simulink model "Lab07B"  (R2021a)
settings: Solver=VariableStepAuto  StartTime=0.0  StopTime=50  RelTol=1e-3
undefined symbols (not defined in the file or in its folder): Kh, Kv
libraries: simulink x1
settings Model: Creator=levivandek  LastModifiedBy=levivandek

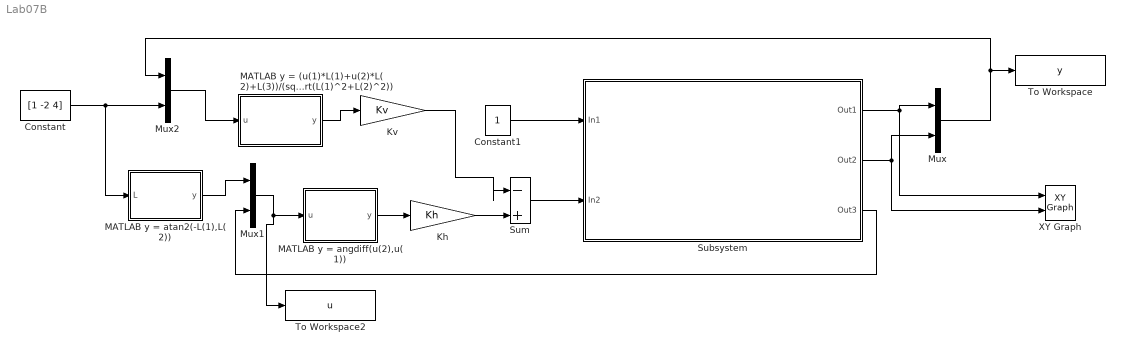
== system Lab07B ==
  Constant : Constant  Value=[1 -2 4]
  Constant1 : Constant
  Kh : Gain  Gain=Kh
  Kv : Gain  Gain=Kv
  MATLAB y = (u(1)*L(1)+u(2)*L(2)+L(3))/(sqrt(L(1)^2+L(2)^2)) : MATLAB Function  TreatAsAtomicUnit=on
  MATLAB y = angdiff(u(2),u(1)) : MATLAB Function  TreatAsAtomicUnit=on
  MATLAB y = atan2(-L(1),L(2)) : MATLAB Function  TreatAsAtomicUnit=on
  Mux : Mux  Inputs=2
  Mux1 : Mux  Inputs=2
  Mux2 : Mux  Inputs=2
  Subsystem : Subsystem
  Sum : Sum  Inputs=|-+
  To Workspace : ToWorkspace  VariableName=y  SaveFormat=Timeseries  SampleTime=-1
  To Workspace2 : ToWorkspace  VariableName=u  SaveFormat=Timeseries  SampleTime=-1
  XY Graph : simulink/Sinks/XY Graph  xmin=-10  xmax=10  ymin=-4  ymax=12  st=-1
  wires:
  Subsystem/2(Out2) -> Mux/2, XY Graph/2
  Subsystem/1(Out1) -> XY Graph/1, Mux/1
  Mux/1 -> Mux2/1, To Workspace/1
  Subsystem/3(Out3) -> Mux1/2
  MATLAB y = angdiff(u(2),u(1))/1(y) -> Kh/1
  Mux1/1 -> To Workspace2/1, MATLAB y = angdiff(u(2),u(1))/1(u)
  MATLAB y = (u(1)*L(1)+u(2)*L(2)+L(3))/(sqrt(L(1)^2+L(2)^2))/1(y) -> Kv/1
  MATLAB y = atan2(-L(1),L(2))/1(y) -> Mux1/1
  Constant/1 -> MATLAB y = atan2(-L(1),L(2))/1(L), Mux2/2
  Kh/1 -> Sum/2
  Kv/1 -> Sum/1
  Sum/1 -> Subsystem/2(In2)
  Constant1/1 -> Subsystem/1(In1)
  Mux2/1 -> MATLAB y = (u(1)*L(1)+u(2)*L(2)+L(3))/(sqrt(L(1)^2+L(2)^2))/1(u)

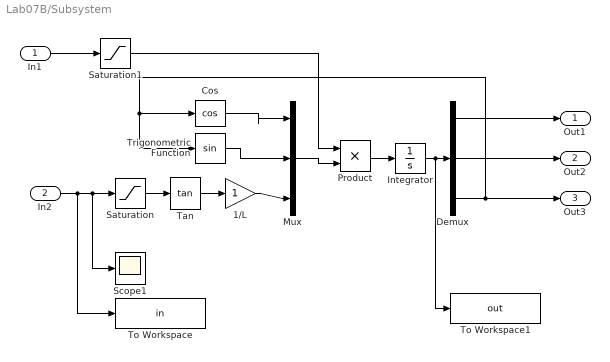
== system Lab07B/Subsystem ==
  In1 : Inport
  In2 : Inport  Port=2
  1/L : Gain
  Cos : Trigonometry  Operator=cos
  Demux : Demux  Outputs=3
  Integrator : Integrator  InitialCondition=[8 5 pi/2]
  Mux : Mux  Inputs=3
  Product : Product
  Saturation : Saturate  UpperLimit=1  LowerLimit=-1
  Saturation1 : Saturate  UpperLimit=1  LowerLimit=-1
  Scope1 : Scope
  Tan : Trigonometry  Operator=tan
  To Workspace : ToWorkspace  VariableName=in  SaveFormat=Timeseries  SampleTime=-1
  To Workspace1 : ToWorkspace  VariableName=out  SaveFormat=Timeseries  SampleTime=-1
  Trigonometric Function : Trigonometry
  Out1 : Outport
  Out2 : Outport  Port=2
  Out3 : Outport  Port=3
  wires:
  Cos/1 -> Mux/1
  Demux/1 -> Out1/1
  In2/1 -> To Workspace/1, Scope1/1, Saturation/1
  1/L/1 -> Mux/3
  Product/1 -> Integrator/1
  Integrator/1 -> To Workspace1/1, Demux/1
  Saturation1/1 -> Product/1
  In1/1 -> Saturation1/1
  Saturation/1 -> Tan/1
  Trigonometric Function/1 -> Mux/2
  Demux/3 -> Out3/1, Cos/1, Trigonometric Function/1
  Demux/2 -> Out2/1
  Mux/1 -> Product/2
  Tan/1 -> 1/L/1

== matlab function Lab07B/MATLAB y = angdiff(u(2),u(1)) ==
  data: u input size=2; y output
function y= fcn(u)
    y = angdiff(u(2), u(1));
end
    
% function y= fcn(beta, alpha)
% 
%     gama=alpha-beta;
% 
%     if abs(gama)>2*pi
%         gama1=gama-fix(gama/2/pi)*2*pi; %removes the decimals
%     else
%         gama1=gama;
%     end
% 
%     if abs(gama1)>pi
%        if gama1>0
%            y=gama1-2*pi;
%        else
%            y=gama1+2*pi;
%        end
%     else
%         y=gama1;
%     end
% 
% end

== matlab function Lab07B/MATLAB y = atan2(-L(1),L(2)) ==
  data: L input; y output
function y = fcn(L)

y = atan2(-L(1),L(2));

== matlab function Lab07B/MATLAB y = (u(1)*L(1)+u(2)*L(2)+L(3))//(sqrt(L(1)^2+L(2)^2)) ==
  data: u input; y output
function y = fcn(u)

y = (u(1)*u(3)+u(2)*u(4)+u(5))/(sqrt(u(3)^2+u(4)^2));
